simulink model "S861a_ST24R_ID_ABBIRB120"  (R2020b)
settings: Solver=FixedStepAuto  StartTime=0.0  StopTime=10  FixedStep=0.0005  RelTol=1e-3  EnableMultiTasking=on
undefined symbols (not defined in the file or in its folder): X, Y, Z
libraries: sm_lib x123, nesl_utility x35, robotcorelib x2
(part 4 of 4)

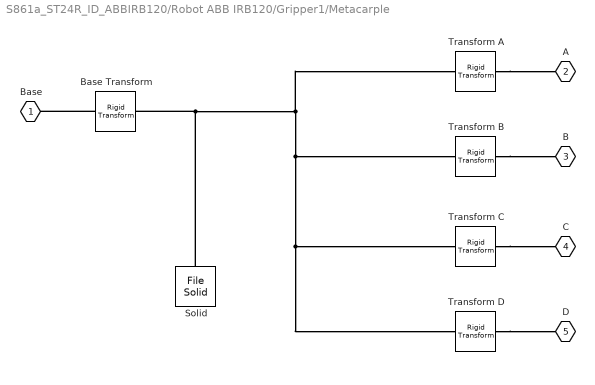
== system S861a_ST24R_ID_ABBIRB120/Robot ABB IRB120/Gripper1/Metacarple ==
  Base Transform : sm_lib/Frames and Transforms/Rigid Transform  TranslationMethod=StandardAxis  TranslationStandardOffset=0.075  TranslationLengthUnit=m  TranslationStandardAxis=+X  TranslationCartesianOffset=[-1.27 0 0]  TranslationROffset=0  TranslationROffsetUnits=m  TranslationZOffset=0  TranslationZOffsetUnits=m  TranslationThetaOffset=0  TranslationThetaOffsetUnits=deg  RotationMethod=RotationSequence  RotationAngleUnits=deg  RotationStandardAxis=+Y  RotationAngle=90  RotationArbitraryAxis=[-1 -1 1]  FollAlignAxisA=+Z  BaseAlignAxisA=+X  FollAlignAxisB=+Y  BaseAlignAxisB=-Y  RotationSequenceAxes=FollowerAxes  RotationSequence=ZYX  RotationSequenceAngles=[90 0 90]  RotationSequenceAnglesUnits=deg  RotationMatrix=[1 0 0; 0 1 0; 0 0 1]
  Solid : sm_lib/Body Elements/File Solid  ExtGeomFileName=sm_srobot_metacarples.step  UnitType=FromFile  ExtGeomFileUnits=cm  StepReaderType=OCC  ExportConvexHullGeometry=off  InertiaType=CalculateFromGeometry  Mass=0.2949697962727843  MassUnits=kg  CenterOfMass=[0.51853214693243821 -2.1099755536633642e-07 1.2556451003194651e-07]  CenterOfMassUnits=cm  MomentsOfInertia=[0.78710657037075882 0.85556914968787445 0.70502786812617768]  MomentsOfInertiaUnits=kg*cm^2  ProductsOfInertia=[-8.2010371922616861e-08 1.5884273115413992e-07 1.1530290569471579e-07]  ProductsOfInertiaUnits=kg*cm^2  BasedOnType=Density  Density=1000  DensityUnits=kg/(m^3)  DoExposeReferenceFrame=on  SerializedFrames=<Frames/>  GraphicType=FromGeometry  MarkerShape=Sphere  MarkerSize=10  MarkerSizeUnits=m  GraphicVisPropType=SimpleVisualProperties  GraphicDiffuseColor=[0.6588235294117647 1 0.82745098039215681]  GraphicSpecularColor=[0.5 0.5 0.5 1.0]  GraphicAmbientColor=[0.15 0.15 0.15 1.0]  GraphicEmissiveColor=[0.0 0.0 0.0 1.0]  GraphicShininess=75  GraphicOpacity=1
  Transform A : sm_lib/Frames and Transforms/Rigid Transform  TranslationMethod=Cartesian  TranslationStandardOffset=0  TranslationLengthUnit=cm  TranslationStandardAxis=+Z  TranslationCartesianOffset=[1.6022 -0.91801024484276572 -1.1156]  TranslationROffset=0  TranslationROffsetUnits=m  TranslationZOffset=0  TranslationZOffsetUnits=m  TranslationThetaOffset=0  TranslationThetaOffsetUnits=deg  RotationMethod=ArbitraryAxis  RotationAngleUnits=deg  RotationStandardAxis=+Z  RotationAngle=120  RotationArbitraryAxis=[-1 -1 -1]  FollAlignAxisA=+X  BaseAlignAxisA=+Y  FollAlignAxisB=+Y  BaseAlignAxisB=+Z  RotationSequenceAxes=FollowerAxes  RotationSequence=XYX  RotationSequenceAngles=[0 0 0]  RotationSequenceAnglesUnits=deg  RotationMatrix=[1 0 0; 0 1 0; 0 0 1]
  Transform B : sm_lib/Frames and Transforms/Rigid Transform  TranslationMethod=Cartesian  TranslationStandardOffset=0  TranslationLengthUnit=cm  TranslationStandardAxis=+Z  TranslationCartesianOffset=[3.6475045256124723 -0.9180102448427655 -0.54883545692650082]  TranslationROffset=0  TranslationROffsetUnits=m  TranslationZOffset=0  TranslationZOffsetUnits=m  TranslationThetaOffset=0  TranslationThetaOffsetUnits=deg  RotationMethod=ArbitraryAxis  RotationAngleUnits=deg  RotationStandardAxis=+Z  RotationAngle=120  RotationArbitraryAxis=[-1 -1 -1]  FollAlignAxisA=+X  BaseAlignAxisA=+Y  FollAlignAxisB=+Y  BaseAlignAxisB=+Z  RotationSequenceAxes=FollowerAxes  RotationSequence=XYX  RotationSequenceAngles=[0 0 0]  RotationSequenceAnglesUnits=deg  RotationMatrix=[1 0 0; 0 1 0; 0 0 1]
  Transform C : sm_lib/Frames and Transforms/Rigid Transform  TranslationMethod=Cartesian  TranslationStandardOffset=0  TranslationLengthUnit=cm  TranslationStandardAxis=+Z  TranslationCartesianOffset=[3.6475045256124723 -0.9180102448427655 0.54883545692650082]  TranslationROffset=0  TranslationROffsetUnits=m  TranslationZOffset=0  TranslationZOffsetUnits=m  TranslationThetaOffset=0  TranslationThetaOffsetUnits=deg  RotationMethod=ArbitraryAxis  RotationAngleUnits=deg  RotationStandardAxis=+Z  RotationAngle=120  RotationArbitraryAxis=[-1 -1 -1]  FollAlignAxisA=+X  BaseAlignAxisA=+Y  FollAlignAxisB=+Y  BaseAlignAxisB=+Z  RotationSequenceAxes=FollowerAxes  RotationSequence=XYX  RotationSequenceAngles=[0 0 0]  RotationSequenceAnglesUnits=deg  RotationMatrix=[1 0 0; 0 1 0; 0 0 1]
  Transform D : sm_lib/Frames and Transforms/Rigid Transform  TranslationMethod=Cartesian  TranslationStandardOffset=0  TranslationLengthUnit=cm  TranslationStandardAxis=+Z  TranslationCartesianOffset=[1.6022 -0.91801024484276572 1.1156]  TranslationROffset=0  TranslationROffsetUnits=m  TranslationZOffset=0  TranslationZOffsetUnits=m  TranslationThetaOffset=0  TranslationThetaOffsetUnits=deg  RotationMethod=ArbitraryAxis  RotationAngleUnits=deg  RotationStandardAxis=+Z  RotationAngle=120  RotationArbitraryAxis=[-1 -1 -1]  FollAlignAxisA=+X  BaseAlignAxisA=+Y  FollAlignAxisB=+Y  BaseAlignAxisB=+Z  RotationSequenceAxes=FollowerAxes  RotationSequence=XYX  RotationSequenceAngles=[0 0 0]  RotationSequenceAnglesUnits=deg  RotationMatrix=[1 0 0; 0 1 0; 0 0 1]
  Base : PMIOPort  Side=Left
  A : PMIOPort  Port=2  Side=Right
  B : PMIOPort  Port=3  Side=Right
  C : PMIOPort  Port=4  Side=Right
  D : PMIOPort  Port=5  Side=Right
  connections:
  Solid/RConn1 -- Base Transform/LConn1 -- Transform D/LConn1 -- Transform C/LConn1 -- Transform B/LConn1 -- Transform A/LConn1
  Transform D/RConn1 -- D/RConn1
  Transform C/RConn1 -- C/RConn1
  Transform B/RConn1 -- B/RConn1
  Transform A/RConn1 -- A/RConn1
  Base Transform/RConn1 -- Base/RConn1

== system S861a_ST24R_ID_ABBIRB120/Robot ABB IRB120/Gripper1/Right Finger Tips ==
  Solid : sm_lib/Body Elements/File Solid  ExtGeomFileName=sm_srobot_fingertips.step  UnitType=FromFile  ExtGeomFileUnits=cm  StepReaderType=OCC  ExportConvexHullGeometry=off  InertiaType=CalculateFromGeometry  Mass=0.025178123679146753  MassUnits=kg  CenterOfMass=[0.28569571896451468 -5.4578424046040067e-05 0.069036811438125095]  CenterOfMassUnits=cm  MomentsOfInertia=[0.0065444380491917675 0.049015093978220708 0.046494149823922123]  MomentsOfInertiaUnits=kg*cm^2  ProductsOfInertia=[1.4396383276680692e-06 0.01060495039373101 -3.3718497055589141e-06]  ProductsOfInertiaUnits=kg*cm^2  BasedOnType=Density  Density=1000  DensityUnits=kg/(m^3)  DoExposeReferenceFrame=on  SerializedFrames=<Frames/>  GraphicType=FromGeometry  MarkerShape=Sphere  MarkerSize=10  MarkerSizeUnits=m  GraphicVisPropType=SimpleVisualProperties  GraphicDiffuseColor=[0.47450980392156861 0.73725490196078436 1]  GraphicSpecularColor=[0.5 0.5 0.5 1.0]  GraphicAmbientColor=[0.15 0.15 0.15 1.0]  GraphicEmissiveColor=[0.0 0.0 0.0 1.0]  GraphicShininess=75  GraphicOpacity=1
  Transform to First : sm_lib/Frames and Transforms/Rigid Transform  TranslationMethod=Cartesian  TranslationStandardOffset=0  TranslationLengthUnit=cm  TranslationStandardAxis=+Z  TranslationCartesianOffset=[-2.544215292032415 -0.74021024484276632 0.82666565983828855]  TranslationROffset=0  TranslationROffsetUnits=m  TranslationZOffset=0  TranslationZOffsetUnits=m  TranslationThetaOffset=0  TranslationThetaOffsetUnits=deg  RotationMethod=ArbitraryAxis  RotationAngleUnits=deg  RotationStandardAxis=+Z  RotationAngle=120  RotationArbitraryAxis=[-1 -1 -1]  FollAlignAxisA=+X  BaseAlignAxisA=+Y  FollAlignAxisB=+Y  BaseAlignAxisB=+Z  RotationSequenceAxes=FollowerAxes  RotationSequence=XYX  RotationSequenceAngles=[0 0 0]  RotationSequenceAnglesUnits=deg  RotationMatrix=[1 0 0; 0 1 0; 0 0 1]
  Transform to Second : sm_lib/Frames and Transforms/Rigid Transform  TranslationMethod=Cartesian  TranslationStandardOffset=0  TranslationLengthUnit=cm  TranslationStandardAxis=+Z  TranslationCartesianOffset=[-0.508 0.61321024484276621 -0.2032]  TranslationROffset=0  TranslationROffsetUnits=m  TranslationZOffset=0  TranslationZOffsetUnits=m  TranslationThetaOffset=0  TranslationThetaOffsetUnits=deg  RotationMethod=ArbitraryAxis  RotationAngleUnits=deg  RotationStandardAxis=+Z  RotationAngle=120  RotationArbitraryAxis=[1 -1 1]  FollAlignAxisA=+X  BaseAlignAxisA=+Y  FollAlignAxisB=+Y  BaseAlignAxisB=+Z  RotationSequenceAxes=FollowerAxes  RotationSequence=XYX  RotationSequenceAngles=[0 0 0]  RotationSequenceAnglesUnits=deg  RotationMatrix=[1 0 0; 0 1 0; 0 0 1]
  Second : PMIOPort  Side=Left
  First : PMIOPort  Port=2  Side=Left
  connections:
  Solid/RConn1 -- Transform to Second/LConn1 -- Transform to First/LConn1
  Transform to First/RConn1 -- First/RConn1
  Transform to Second/RConn1 -- Second/RConn1

== system S861a_ST24R_ID_ABBIRB120/Robot ABB IRB120/Gripper1/Right First Finger Link ==
  Base Transform : sm_lib/Frames and Transforms/Rigid Transform  TranslationMethod=Cartesian  TranslationStandardOffset=0  TranslationLengthUnit=cm  TranslationStandardAxis=+Z  TranslationCartesianOffset=[0 -0.91801024484276572 0]  TranslationROffset=0  TranslationROffsetUnits=m  TranslationZOffset=0  TranslationZOffsetUnits=m  TranslationThetaOffset=0  TranslationThetaOffsetUnits=deg  RotationMethod=ArbitraryAxis  RotationAngleUnits=deg  RotationStandardAxis=+Z  RotationAngle=120  RotationArbitraryAxis=[-1 -1 -1]  FollAlignAxisA=+X  BaseAlignAxisA=+Y  FollAlignAxisB=+Y  BaseAlignAxisB=+Z  RotationSequenceAxes=FollowerAxes  RotationSequence=XYX  RotationSequenceAngles=[0 0 0]  RotationSequenceAnglesUnits=deg  RotationMatrix=[1 0 0; 0 1 0; 0 0 1]
  Follower Transform : sm_lib/Frames and Transforms/Rigid Transform  TranslationMethod=Cartesian  TranslationStandardOffset=0  TranslationLengthUnit=cm  TranslationStandardAxis=+Z  TranslationCartesianOffset=[1.778 -0.74021024484276632 0.381]  TranslationROffset=0  TranslationROffsetUnits=m  TranslationZOffset=0  TranslationZOffsetUnits=m  TranslationThetaOffset=0  TranslationThetaOffsetUnits=deg  RotationMethod=ArbitraryAxis  RotationAngleUnits=deg  RotationStandardAxis=+Z  RotationAngle=120  RotationArbitraryAxis=[-1 -1 -1]  FollAlignAxisA=+X  BaseAlignAxisA=+Y  FollAlignAxisB=+Y  BaseAlignAxisB=+Z  RotationSequenceAxes=FollowerAxes  RotationSequence=XYX  RotationSequenceAngles=[0 0 0]  RotationSequenceAnglesUnits=deg  RotationMatrix=[1 0 0; 0 1 0; 0 0 1]
  Solid : sm_lib/Body Elements/File Solid  ExtGeomFileName=sm_srobot_rfirstfingerlink.step  UnitType=FromFile  ExtGeomFileUnits=cm  StepReaderType=OCC  ExportConvexHullGeometry=off  InertiaType=CalculateFromGeometry  Mass=0.0072753633395043153  MassUnits=kg  CenterOfMass=[0.5793957104083951 -0.065568525374514061 0.41045924650847537]  CenterOfMassUnits=cm  MomentsOfInertia=[0.0013879360712697633 0.0054293297573781941 0.0057606953913205416]  MomentsOfInertiaUnits=kg*cm^2  ProductsOfInertia=[-9.6988344798463436e-05 -0.00030548455416942526 -0.00028825710364633017]  ProductsOfInertiaUnits=kg*cm^2  BasedOnType=Density  Density=1000  DensityUnits=kg/(m^3)  DoExposeReferenceFrame=on  SerializedFrames=<Frames/>  GraphicType=FromGeometry  MarkerShape=Sphere  MarkerSize=10  MarkerSizeUnits=m  GraphicVisPropType=SimpleVisualProperties  GraphicDiffuseColor=[1 1 0.5490196078431373]  GraphicSpecularColor=[0.5 0.5 0.5 1.0]  GraphicAmbientColor=[0.15 0.15 0.15 1.0]  GraphicEmissiveColor=[0.0 0.0 0.0 1.0]  GraphicShininess=75  GraphicOpacity=1
  B : PMIOPort  Side=Left
  F : PMIOPort  Port=2  Side=Right
  connections:
  Solid/RConn1 -- Base Transform/LConn1 -- Follower Transform/LConn1
  Base Transform/RConn1 -- B/RConn1
  Follower Transform/RConn1 -- F/RConn1

== system S861a_ST24R_ID_ABBIRB120/Robot ABB IRB120/Gripper1/Right Second Finger Link ==
  Base Transform : sm_lib/Frames and Transforms/Rigid Transform  TranslationMethod=Cartesian  TranslationStandardOffset=0  TranslationLengthUnit=cm  TranslationStandardAxis=+Z  TranslationCartesianOffset=[2.1844 -0.91801024484276539 0]  TranslationROffset=0  TranslationROffsetUnits=m  TranslationZOffset=0  TranslationZOffsetUnits=m  TranslationThetaOffset=0  TranslationThetaOffsetUnits=deg  RotationMethod=ArbitraryAxis  RotationAngleUnits=deg  RotationStandardAxis=+Z  RotationAngle=120  RotationArbitraryAxis=[-1 -1 -1]  FollAlignAxisA=+X  BaseAlignAxisA=+Y  FollAlignAxisB=+Y  BaseAlignAxisB=+Z  RotationSequenceAxes=FollowerAxes  RotationSequence=XYX  RotationSequenceAngles=[0 0 0]  RotationSequenceAnglesUnits=deg  RotationMatrix=[1 0 0; 0 1 0; 0 0 1]
  Follower Transform : sm_lib/Frames and Transforms/Rigid Transform  TranslationMethod=Cartesian  TranslationStandardOffset=0  TranslationLengthUnit=cm  TranslationStandardAxis=+Z  TranslationCartesianOffset=[0 0.61321024484276621 0]  TranslationROffset=0  TranslationROffsetUnits=m  TranslationZOffset=0  TranslationZOffsetUnits=m  TranslationThetaOffset=0  TranslationThetaOffsetUnits=deg  RotationMethod=ArbitraryAxis  RotationAngleUnits=deg  RotationStandardAxis=+Z  RotationAngle=120  RotationArbitraryAxis=[1 -1 1]  FollAlignAxisA=+X  BaseAlignAxisA=+Y  FollAlignAxisB=+Y  BaseAlignAxisB=+Z  RotationSequenceAxes=FollowerAxes  RotationSequence=XYX  RotationSequenceAngles=[0 0 0]  RotationSequenceAnglesUnits=deg  RotationMatrix=[1 0 0; 0 1 0; 0 0 1]
  Solid : sm_lib/Body Elements/File Solid  ExtGeomFileName=sm_srobot_secondfingerlink.step  UnitType=FromFile  ExtGeomFileUnits=cm  StepReaderType=OCC  ExportConvexHullGeometry=off  InertiaType=CalculateFromGeometry  Mass=0.005347817964666832  MassUnits=kg  CenterOfMass=[1.3095387695944416 0 0]  CenterOfMassUnits=cm  MomentsOfInertia=[0.00062632050801362594 0.0042402045040431545 0.0044495724115703027]  MomentsOfInertiaUnits=kg*cm^2  ProductsOfInertia=[0 0 0]  ProductsOfInertiaUnits=kg*cm^2  BasedOnType=Density  Density=1000  DensityUnits=kg/(m^3)  DoExposeReferenceFrame=on  SerializedFrames=<Frames/>  GraphicType=FromGeometry  MarkerShape=Sphere  MarkerSize=10  MarkerSizeUnits=m  GraphicVisPropType=SimpleVisualProperties  GraphicDiffuseColor=[1 0 0]  GraphicSpecularColor=[0.5 0.5 0.5 1.0]  GraphicAmbientColor=[0.15 0.15 0.15 1.0]  GraphicEmissiveColor=[0.0 0.0 0.0 1.0]  GraphicShininess=75  GraphicOpacity=1
  B : PMIOPort  Side=Left
  F : PMIOPort  Port=2  Side=Right
  connections:
  Solid/RConn1 -- Follower Transform/LConn1 -- Base Transform/LConn1
  Base Transform/RConn1 -- B/RConn1
  Follower Transform/RConn1 -- F/RConn1
